simulink model "simulink_ompc_discrete"  (R2022b)
settings: Solver=ode8  StartTime=0.0  StopTime=time  FixedStep=Ts  RelTol=1e-3
values from neighbouring files (symbols this model uses):
  A_bar = [Ad, Z_unknown; zeros(n_disturbances, n_states), zeros(n_disturbances)]    [plik_generujDane.m]
  B_bar = [Bd; zeros(n_disturbances, size(Bd, 2))]    [plik_generujDane.m]
  Bd = Bd(:, 1:size(B, 2))    [plik_generujDane.m]
  C_bar = [C_measured, zeros(size(C_measured, 1), n_disturbances)]    [plik_generujDane.m]
  C_measured = create_Cobserver_matrix(C, N)    [plik_generujDane.m]
  D = Dm    [generateBuilding.m]    (also in generateFloor.m)
  Kz = zeros(ny * na, nd * na)    [create_Kz_matrix.m]    (also in ompc_cost.m = [-K, eye(nu), zeros(nu,(nc-1)*nu), [K*Kxr+Kur,zeros(nu,ny*(n)
  L = vecNeighbors(1,1)    [genRoomParams.m]    (also in plik_generujDane.m = L')
  na = 36    [plik_generujDane.m]
  nc = 108    [plik_generujDane.m]
  npred = 108    [plik_generujDane.m]
  Sc = Spsi(nx+1:nx+nuc, nx+1:nx+nuc)    [ompc_cost.m]
  Scr = Spsi(nx+1:nx+nuc, nx+nuc+1:end)    [ompc_cost.m]
  Sxc = Spsi(1:nx, nx+1:nx+nuc)    [ompc_cost.m]
  time = 3600*24    (= 86400)    [plik_generujDane.m]
  trajDist = [trajDist;zeros(nz-size(trajDist,1),size(trajDist,2))]    [plik_generujDane.m]
  trajRef = [21 21 21 21 21 ... (first row only)    [plik_generujDane.m]
  Ts = 720    [plik_generujDane.m]
  umax = 40*ones(nu,1)    [plik_generujDane.m]
  umin = 20*ones(nu,1)    [plik_generujDane.m]
  xmax = xmax'    [plik_generujDane.m]
  xmin = xmin'    [plik_generujDane.m]
  ymax = Ta_max*ones(ny,1)    [plik_generujDane.m]
  ymin = Ta_min*ones(ny,1)    [plik_generujDane.m]
  Z = [Z zeros(nZ, nZmcol-3); Zm(:,1:2) zeros(nZm, nZcol-3) Zm(:,3:end)]    [generateBuilding.m]    (also in generateFloor.m = [Z zeros(nZ,1); Zm(:,1:3) zeros(nZm,nZcol-3) Zm(:,4)]; mergeFloorModels.m = Z0)
  Z_bar_known = [Z_known; zeros(n_disturbances, size(Z_known, 2))]    [plik_generujDane.m]
  Zd = Bd(:, size(B,2)+1:end)    [plik_generujDane.m]
undefined symbols (not defined in the file or in its folder): Ad, Ao, Bo, Cd, Co, Go, K, x0
libraries: eeStairGenerator x1, simulink x1
settings Model: Creator=artur  LastModifiedBy=artur

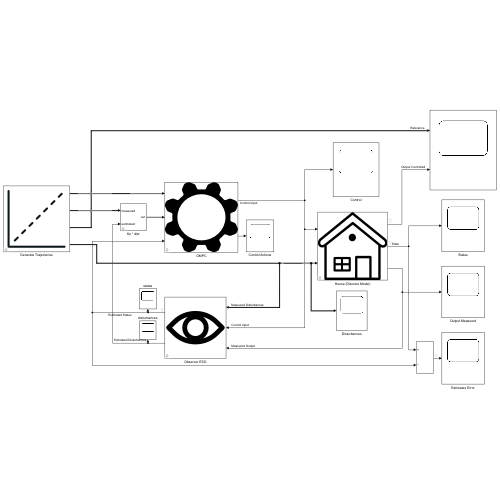
[thumbnail: Simulink's stored preview of the top-level diagram]
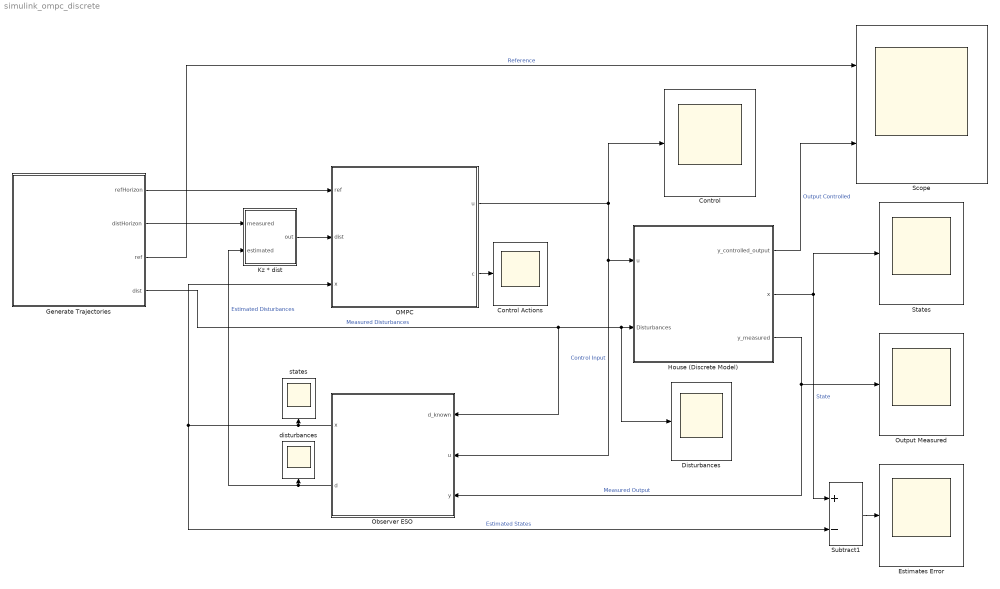
== system simulink_ompc_discrete ==
  Control : Scope
  Control Actions : Scope
  Disturbances : Scope
  Estimates Error : Scope
  Generate Trajectories : Subsystem  mask{time=time, Ts=Ts, na=na, refValues=trajRef, distValues=trajDist}
      mask prompts: time "Czas symulacji"; Ts "Okres próbkowania"; na "Horyzont trajektorii"; refValues "Trajektoria referencyjna"; distValues "Trajektoria zakłóceń"
      mask Display: image('C:\Users\artur\OneDrive\Dokumenty\MATLAB\Magisterka\model\images\plot-icon.svg'); % Use "Edit Image" on toolstrip to change.
  House (Discrete Model) : Subsystem  mask{A=Ad, B=Bd, C=Cd, C_measured=C_measured, D=D, Z=Zd, x0=x0}
      mask prompts: A "Macierz A:"; B "Macierz B"; C "Macierz C sterowane"; C_measured "Macierz C mierzone"; D "Macierz D"; Z "Macierz zakłóceń Z"; x0 "War. początkowe"
      mask DialogControl ParameterGroupVar Prompt: Parametry modelu
      mask Display: image('C:\Users\artur\OneDrive\Dokumenty\MATLAB\Magisterka\model\images\house-icon.svg'); % Use "Edit Image" on toolstrip to change.
  Kz * dist : Subsystem  mask{Ad=Ad, Cd=Cd, Zd=Zd, na=na}
      mask prompts: Ad "A"; Cd "C"; Zd "Z"
  OMPC : Subsystem  mask{A=Ad, B=Bd, C=Cd, nc=nc, npred=npred, na=na, Sxc=Sxc, Scr=Scr, Sc=Sc, K=K, umax=umax, umin=umin, ymax=ymax, ymin=ymin, xmax=xmax, xmin=xmin}
      mask prompts: A "Macierz A"; B "Macierz  B"; C "Macierz C"; nc "Liczba zmiennych decyzyjnych"; npred "Horyzont predykcji"; na "Horyzont trajektorii"; Sxc "Macierz Sxc"; Scr "Macierz Scr"; Sc "Macierz Sc"; K "Macierz K"
      mask DialogControl ParameterGroupVar Prompt: Parametry modelu
      mask DialogControl Container3 Prompt: Parametry regulatora
      mask DialogControl Container4 Prompt: Ograniczenia
      mask Display: image('C:\Users\artur\OneDrive\Dokumenty\MATLAB\Magisterka\model\images\cogwheel-icon.svg'); % Use "Edit Image" on toolstrip to change.
  Observer ESO : Subsystem  mask{A_bar=A_bar, B_bar=B_bar, C_bar=C_bar, A=Ad, L=L, Z_bar_known=Z_bar_known}
      mask DialogControl Observer Prompt: Parametry Obserwatora
      mask Display: image('C:\Users\artur\OneDrive\Dokumenty\MATLAB\Magisterka\model\images\eye-icon.svg'); % Use "Edit Image" on toolstrip to change.
  Output Measured : Scope
  Scope : Scope  NumInputPorts=2
  States : Scope
  Subtract1 : Sum  Inputs=+-
  disturbances : Scope
  states : Scope
  wires:
  Observer ESO/1(x) -> OMPC/3(x), Subtract1/2, states/1  "Estimated States"
  OMPC/1(u) -> House (Discrete Model)/1(u), Observer ESO/2(u), Control/1  "Control Input"
  House (Discrete Model)/2(x) -> States/1, Subtract1/1  "State"
  Generate Trajectories/3(ref) -> Scope/1  "Reference"
  Generate Trajectories/1(refHorizon) -> OMPC/1(ref)
  House (Discrete Model)/3(y_measured) -> Output Measured/1, Observer ESO/3(y)  "Measured Output"
  Observer ESO/2(d) -> disturbances/1, Kz * dist/2(estimated)  "Estimated Disturbances"
  House (Discrete Model)/1(y_controlled_output) -> Scope/2  "Output Controlled"
  Kz * dist/1(out) -> OMPC/2(dist)
  Generate Trajectories/2(distHorizon) -> Kz * dist/1(measured)
  Subtract1/1 -> Estimates Error/1
  OMPC/2(c) -> Control Actions/1
  Generate Trajectories/4(dist) -> Observer ESO/1(d_known), House (Discrete Model)/2(Disturbances), Disturbances/1  "Measured Disturbances"

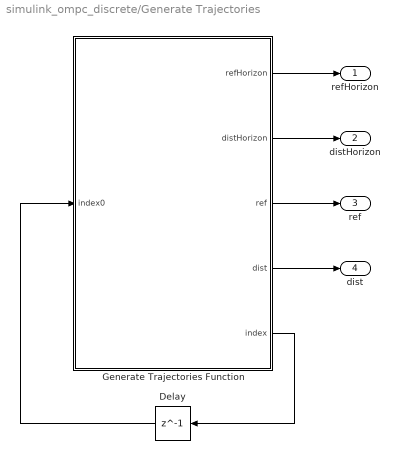
== system simulink_ompc_discrete/Generate Trajectories ==
  Delay : Delay  DelayLength=1  InitialCondition=1
  Generate Trajectories Function : MATLAB Function  TreatAsAtomicUnit=on
  refHorizon : Outport
  distHorizon : Outport  Port=2
  ref : Outport  Port=3
  dist : Outport  Port=4
  wires:
  Generate Trajectories Function/2(distHorizon) -> distHorizon/1
  Generate Trajectories Function/3(ref) -> ref/1
  Generate Trajectories Function/1(refHorizon) -> refHorizon/1
  Generate Trajectories Function/5(index) -> Delay/1
  Delay/1 -> Generate Trajectories Function/1(index0)
  Generate Trajectories Function/4(dist) -> dist/1

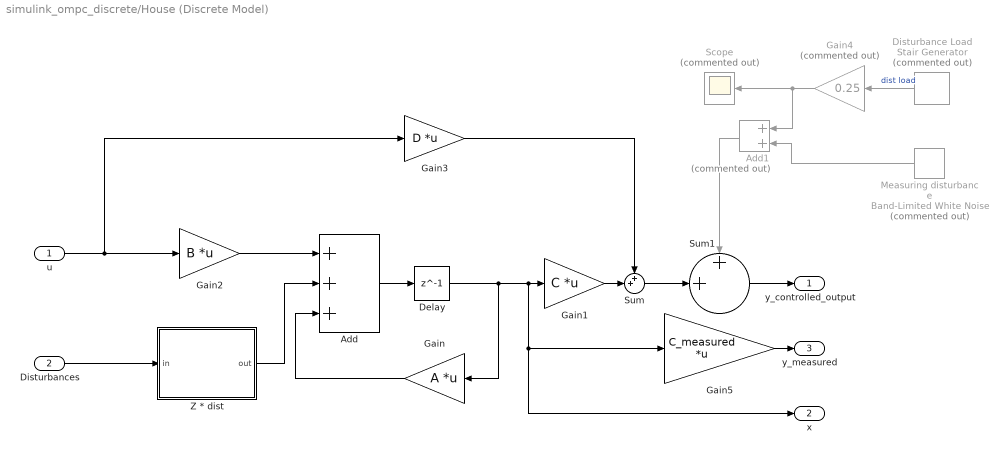
== system simulink_ompc_discrete/House (Discrete Model) ==
  u : Inport
  Disturbances : Inport  Port=2
  Add : Sum  Inputs=+++
  Add1 : Sum  Commented=on
  Delay : Delay  DelayLength=1  InitialCondition=x0
  Disturbance Load : eeStairGenerator/Stair Generator  Commented=on  LabelModeActiveChoice=Discrete  TimeInput=[0 5 10 15 20 25 30 35 40 45 50]  AmplitudeInput=[1 1 1 -1 -1 -1 1 1 -1 -1 1]  SampleTime=0.1  RepeatPattern=on  OutDataTypeStr=double
      settings: LibrarySourceBlock=ee_sl_lib/General Control/Stair Generator
  Gain : Gain  Gain=A  Multiplication=Matrix(K*u) (u vector)
  Gain1 : Gain  Gain=C  Multiplication=Matrix(K*u) (u vector)
  Gain2 : Gain  Gain=B  Multiplication=Matrix(K*u) (u vector)
  Gain3 : Gain  Gain=D  Multiplication=Matrix(K*u)
  Gain4 : Gain  Commented=on  Gain=0.25
  Gain5 : Gain  Gain=C_measured  Multiplication=Matrix(K*u) (u vector)
  Measuring disturbance : simulink/Sources/Band-Limited White Noise  Commented=on  Cov=[0.002]  Ts=0.1  seed=[23341]
  Scope : Scope  Commented=on
  Sum : Sum  Inputs=++|
  Sum1 : Sum  Inputs=++|
  Z * dist : Subsystem  mask{Z=Z}
  y_controlled_output : Outport
  x : Outport  Port=2
  y_measured : Outport  Port=3
  wires:
  u/1 -> Gain3/1, Gain2/1
  Delay/1 -> Gain5/1, x/1, Gain1/1, Gain/1
  Add/1 -> Delay/1
  Gain2/1 -> Add/1
  Gain1/1 -> Sum/2
  Gain3/1 -> Sum/1
  Sum1/1 -> y_controlled_output/1
  Sum/1 -> Sum1/2
  Disturbance Load/1 -> Gain4/1  "dist load"
  Add1/1 -> Sum1/1
  Measuring disturbance/1 -> Add1/2
  Gain4/1 -> Add1/1, Scope/1
  Gain/1 -> Add/3
  Disturbances/1 -> Z * dist/1(in)
  Z * dist/1(out) -> Add/2
  Gain5/1 -> y_measured/1

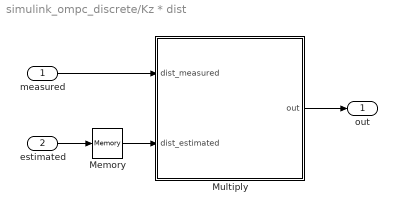
== system simulink_ompc_discrete/Kz * dist ==
  measured : Inport
  estimated : Inport  Port=2
  Memory : Memory  InitialCondition=zeros(size(Z,2)-3,1)
  Multiply : MATLAB Function  TreatAsAtomicUnit=on
  out : Outport
  wires:
  Multiply/1(out) -> out/1
  measured/1 -> Multiply/1(dist_measured)
  estimated/1 -> Memory/1
  Memory/1 -> Multiply/2(dist_estimated)

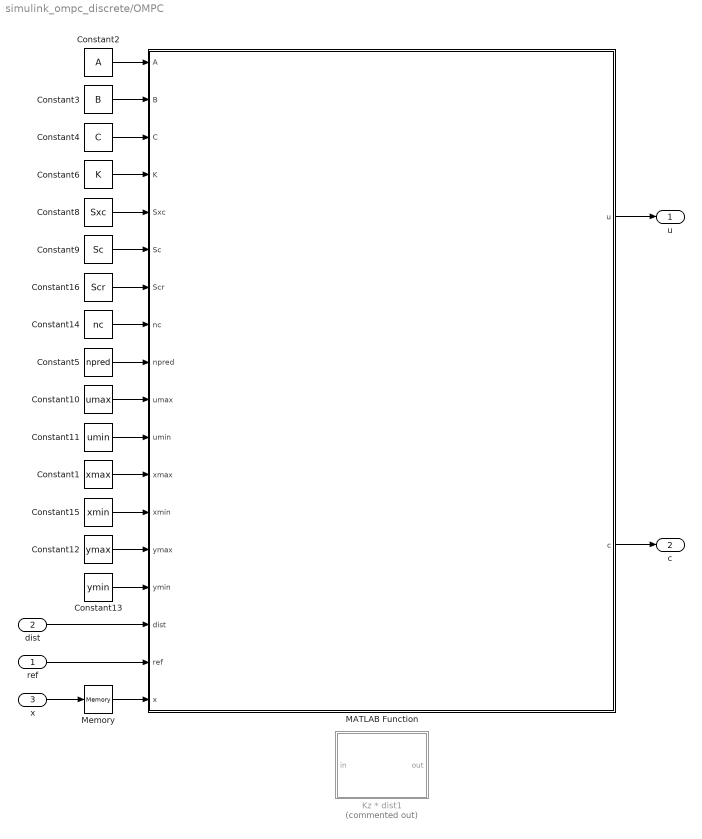
== system simulink_ompc_discrete/OMPC ==
  ref : Inport
  dist : Inport  Port=2
  x : Inport  Port=3
  Constant1 : Constant  Value=xmax  VectorParams1D=off
  Constant10 : Constant  Value=umax  VectorParams1D=off
  Constant11 : Constant  Value=umin  VectorParams1D=off
  Constant12 : Constant  Value=ymax
  Constant13 : Constant  Value=ymin
  Constant14 : Constant  Value=nc
  Constant15 : Constant  Value=xmin
  Constant16 : Constant  Value=Scr  VectorParams1D=off
  Constant2 : Constant  Value=A
  Constant3 : Constant  Value=B  VectorParams1D=off
  Constant4 : Constant  Value=C  VectorParams1D=off
  Constant5 : Constant  Value=npred
  Constant6 : Constant  Value=K  VectorParams1D=off
  Constant8 : Constant  Value=Sxc  VectorParams1D=off
  Constant9 : Constant  Value=Sc  VectorParams1D=off
  Kz * dist1 : Subsystem  Commented=on  mask{Kz=Kz}
  MATLAB Function : MATLAB Function  TreatAsAtomicUnit=on
  Memory : Memory  InitialCondition=x0
  u : Outport
  c : Outport  Port=2
  wires:
  Constant6/1 -> MATLAB Function/4(K)
  Constant9/1 -> MATLAB Function/6(Sc)
  Constant8/1 -> MATLAB Function/5(Sxc)
  Constant2/1 -> MATLAB Function/1(A)
  Constant4/1 -> MATLAB Function/3(C)
  x/1 -> Memory/1
  Constant3/1 -> MATLAB Function/2(B)
  ref/1 -> MATLAB Function/17(ref)
  Constant10/1 -> MATLAB Function/10(umax)
  Constant11/1 -> MATLAB Function/11(umin)
  Constant12/1 -> MATLAB Function/14(ymax)
  Constant13/1 -> MATLAB Function/15(ymin)
  Memory/1 -> MATLAB Function/18(x)
  MATLAB Function/2(c) -> c/1
  Constant5/1 -> MATLAB Function/9(npred)
  Constant14/1 -> MATLAB Function/8(nc)
  dist/1 -> MATLAB Function/16(dist)
  Constant15/1 -> MATLAB Function/13(xmin)
  Constant1/1 -> MATLAB Function/12(xmax)
  MATLAB Function/1(u) -> u/1
  Constant16/1 -> MATLAB Function/7(Scr)

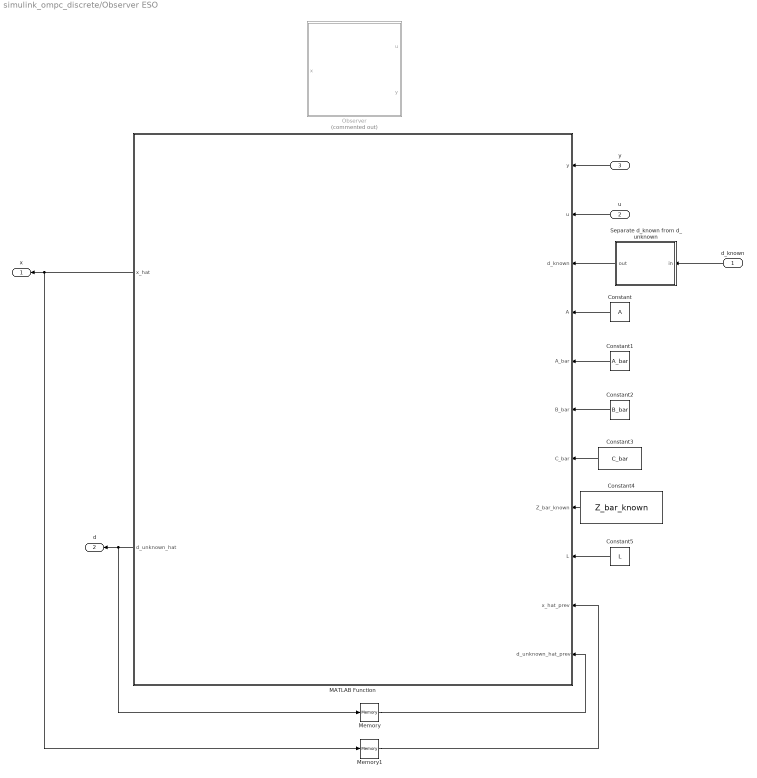
== system simulink_ompc_discrete/Observer ESO ==
  d_known : Inport
  u : Inport  Port=2
  y : Inport  Port=3
  Constant : Constant  Value=A
  Constant1 : Constant  Value=A_bar
  Constant2 : Constant  Value=B_bar
  Constant3 : Constant  Value=C_bar
  Constant4 : Constant  Value=Z_bar_known
  Constant5 : Constant  Value=L
  MATLAB Function : MATLAB Function  TreatAsAtomicUnit=on
  Memory : Memory  InitialCondition=zeros(size(Z,2) - size(Z_bar_known,2),1)
  Memory1 : Memory  InitialCondition=x0
  Observer : Subsystem  Commented=on  mask{Ao=Ao, Bo=Bo, Co=Co, Go=Go, A=Ad}
      mask prompts: Ao "Macierz A"; Bo "Macierz B"; Co "Macierz C"; Go "Macierz G"; A "Macierz A modelu"
      mask DialogControl Observer Prompt: Parametry Obserwatora
      mask Display: image('C:\Users\artur\OneDrive\Dokumenty\MATLAB\Magisterka\model\images\eye-icon.svg'); % Use "Edit Image" on toolstrip to change.
  Separate d_known from d_unknown : MATLAB Function  TreatAsAtomicUnit=on
  x : Outport
  d : Outport  Port=2
  wires:
  MATLAB Function/2(d_unknown_hat) -> Memory/1, d/1
  Memory/1 -> MATLAB Function/11(d_unknown_hat_prev)
  Memory1/1 -> MATLAB Function/10(x_hat_prev)
  MATLAB Function/1(x_hat) -> Memory1/1, x/1
  y/1 -> MATLAB Function/1(y)
  u/1 -> MATLAB Function/2(u)
  Constant/1 -> MATLAB Function/4(A)
  Constant1/1 -> MATLAB Function/5(A_bar)
  Constant2/1 -> MATLAB Function/6(B_bar)
  Constant3/1 -> MATLAB Function/7(C_bar)
  Constant4/1 -> MATLAB Function/8(Z_bar_known)
  Constant5/1 -> MATLAB Function/9(L)
  d_known/1 -> Separate d_known from d_unknown/1(in)
  Separate d_known from d_unknown/1(out) -> MATLAB Function/3(d_known)

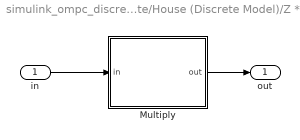
== system simulink_ompc_discrete/House (Discrete Model)/Z * dist ==
  in : Inport
  Multiply : MATLAB Function  TreatAsAtomicUnit=on
  out : Outport
  wires:
  Multiply/1(out) -> out/1
  in/1 -> Multiply/1(in)

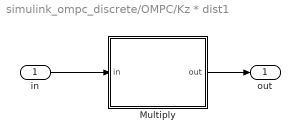
== system simulink_ompc_discrete/OMPC/Kz * dist1 ==
  in : Inport
  Multiply : MATLAB Function  TreatAsAtomicUnit=on
  out : Outport
  wires:
  Multiply/1(out) -> out/1
  in/1 -> Multiply/1(in)

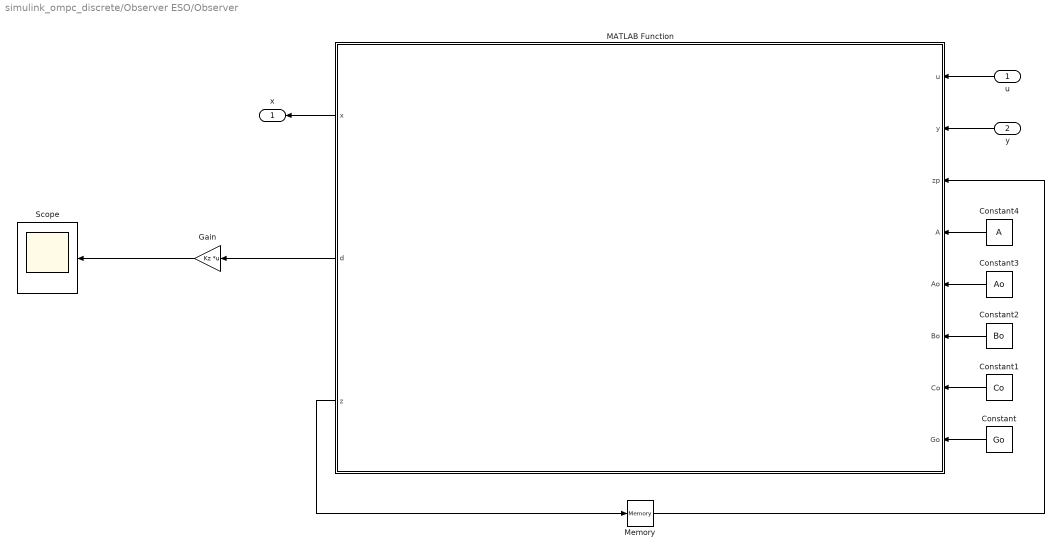
== system simulink_ompc_discrete/Observer ESO/Observer ==
  u : Inport
  y : Inport  Port=2
  Constant : Constant  Value=Go  VectorParams1D=off
  Constant1 : Constant  Value=Co  VectorParams1D=off
  Constant2 : Constant  Value=Bo  VectorParams1D=off
  Constant3 : Constant  Value=Ao  VectorParams1D=off
  Constant4 : Constant  Value=A
  Gain : Gain  Gain=Kz  Multiplication=Matrix(K*u) (u vector)
  MATLAB Function : MATLAB Function  TreatAsAtomicUnit=on
  Memory : Memory  InitialCondition=[x0;zeros(size(Z,2),1)]
  Scope : Scope
  x : Outport
  wires:
  Constant3/1 -> MATLAB Function/5(Ao)
  Constant1/1 -> MATLAB Function/7(Co)
  Constant2/1 -> MATLAB Function/6(Bo)
  Constant/1 -> MATLAB Function/8(Go)
  Memory/1 -> MATLAB Function/3(zp)
  y/1 -> MATLAB Function/2(y)
  u/1 -> MATLAB Function/1(u)
  MATLAB Function/3(z) -> Memory/1
  MATLAB Function/1(x) -> x/1
  Constant4/1 -> MATLAB Function/4(A)
  MATLAB Function/2(d) -> Gain/1
  Gain/1 -> Scope/1

== matlab function simulink_ompc_discrete/Observer ESO/MATLAB Function ==
  data: y input; u input; x_hat output; d_unknown_hat output; d_known input; A input; A_bar input; B_bar input; C_bar input; Z_bar_known input; L input; x_hat_prev input; d_unknown_hat_prev input
function [x_hat, d_unknown_hat] = fcn(y, u, d_known, A, A_bar, B_bar, C_bar, Z_bar_known, L, x_hat_prev, d_unknown_hat_prev)

nx = size(A, 1);

% Rozszerzone stany
x_bar_hat = [x_hat_prev; d_unknown_hat_prev];
y_hat = C_bar * x_bar_hat;

% Aktualizacja estymacji
x_bar_hat = A_bar * x_bar_hat + B_bar * u + Z_bar_known * d_known + L * (y - y_hat);

x_hat = x_bar_hat(1:nx); % Estymowane stany
d_unknown_hat = x_bar_hat(nx+1:end); % Estymowane nieznane zakłócenia
end

== matlab function simulink_ompc_discrete/Observer ESO/Observer/MATLAB Function ==
  data: u input; x output; d output; y input; zp input; A input; Ao input; Bo input; Co input; Go input; z output
function [x,d,z] = fcn(u,y,zp,A,Ao,Bo,Co,Go)

nx = size(A,1);
z = Ao*zp + Bo*u + Go*(y - Co*zp);
x = z(1:nx,:);
d = z(nx+1:end,:);

== matlab function simulink_ompc_discrete/Observer ESO/Separate d_known from d_unknown ==
  data: in input; out output
function out = fcn(in)

out = in(1:3,:);

== matlab function simulink_ompc_discrete/House (Discrete Model)/Z * dist/Multiply ==
  data: in input; out output; Z parameter
function out = fcn(in, Z)
out = Z*in;

== matlab function simulink_ompc_discrete/Generate Trajectories/Generate Trajectories Function ==
  data: refHorizon output size=na*ny; distHorizon output size=na*nz; ref output size=ny; dist output size=nz; time parameter; Ts parameter; na parameter; refValues parameter; distValues parameter; index output; index0 input
function [refHorizon,distHorizon,ref,dist,index] = fcn(time, Ts, na, refValues, distValues, index0)

flag = 1;
[~, refHorizon, ref] = generateTrajectory(refValues,flag,time,Ts,na,index0);
flag = 2;
[~, distHorizon, dist] = generateTrajectory(distValues,flag,time,Ts,na,index0);

index = index0 + 1;

== matlab function simulink_ompc_discrete/Kz * dist/Multiply ==
  data: dist_measured input; dist_estimated input; out output size=ny*na; na parameter; Ad parameter; Cd parameter; Zd parameter
function out = fcn(dist_measured,dist_estimated, na, Ad, Cd, Zd)

%Stwórz macierz kompensacji M
M = create_Kz_matrix(Ad,Cd,Zd,na);

%--------------------------------------------------------------------------
%Stwórz wektor sygnałów zakłócających z danych pomiarowych oraz estymacji
len_measured = length(dist_measured);
len_estimated = length(dist_estimated);
len_repeating = 3 + len_estimated;
num_repeats = len_measured / len_repeating;
disturbance_vector = zeros(size(dist_measured));
idx = 1;
for i = 1:num_repeats
    start_idx = (i-1) * len_repeating + 1;
    disturbance_vector(idx:idx+2) = dist_measured(start_idx:start_idx+2);
    idx = idx + 3;
    disturbance_vector(idx:idx+len_estimated-1) = dist_estimated;
    idx = idx + len_estimated;
end

out = M*disturbance_vector;

== matlab function simulink_ompc_discrete/OMPC/Kz * dist1/Multiply ==
  data: in input; out output; Kz parameter
function out = fcn(in, Kz)
out = Kz*in;

== matlab function simulink_ompc_discrete/OMPC/MATLAB Function ==
  data: A input; B input; C input; K input; Sxc input; Sc input; Scr input; nc input; npred input; umax input; umin input; xmax input; xmin input; ymax input; ymin input; dist input; ref input; x input; u output; c output
function [u,c] = fcn(A,B,C,K,Sxc,Sc,Scr,nc,npred,umax,umin,xmax,xmin,ymax,ymin,dist,ref,x)

[u,ctrl] = ompc_law(A,B,C,K,Sxc,Sc,Scr,umax,umin,xmax,xmin,ymax,ymin,nc,npred,ref,dist,x);
c = ctrl(1:size(B,2),:);
